simulink model "MRAC_Lab2_Normalizado"  (R2020a)
settings: Solver=VariableStepAuto  StartTime=0.0  StopTime=200  RelTol=1e-3
model workspace (MAT data in the model file):
  gamma = Simulink.Parameter
  gamma.Value = 2
  gamma.DataType = 'auto'
  gamma.Dimensions = [1 1]
  gamma2 = Simulink.Parameter
  gamma2.Value = 0.0005
  gamma2.DataType = 'auto'
  gamma2.Dimensions = [1 1]
undefined symbols (not defined in the file): den, num
settings Model: Creator=Lenovo  LastModifiedBy=Lenovo

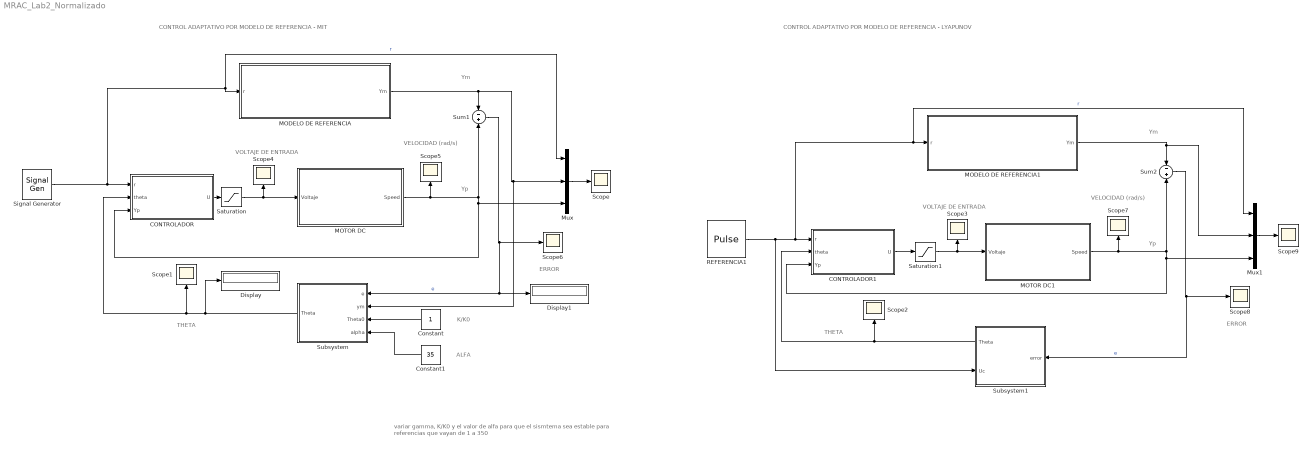
== system MRAC_Lab2_Normalizado ==
  note: variar gamma, K/K0 y el valor de alfa para que el sismtema sea
      | estable para referencias que vayan de 1 a 350
  note: ALFA
  note: K/K0
  note: THETA
  note: VELOCIDAD (rad/s)
  note: Ym
  note: Yp
  note: VOLTAJE DE ENTRADA
  note: ERROR
  note: CONTROL ADAPTATIVO POR MODELO DE REFERENCIA - MIT
  note: THETA
  note: ERROR
  note: Ym
  note: Yp
  note: VELOCIDAD (rad/s)
  note: VOLTAJE DE ENTRADA
  note: CONTROL ADAPTATIVO POR MODELO DE REFERENCIA - LYAPUNOV
  CONTROLADOR : Subsystem
  CONTROLADOR1 : Subsystem
  Constant : Constant
  Constant1 : Constant  Value=35
  Display : Display
  Display1 : Display
  MODELO DE REFERENCIA : Subsystem
  MODELO DE REFERENCIA1 : Subsystem
  MOTOR DC : Subsystem
  MOTOR DC1 : Subsystem
  Mux : Mux  Inputs=3
  Mux1 : Mux  Inputs=3
  REFERENCIA1 : DiscretePulseGenerator  PulseType=Time based  Amplitude=100  Period=20  PulseWidth=50
  Saturation : Saturate  UpperLimit=9  LowerLimit=-9
  Saturation1 : Saturate  UpperLimit=18  LowerLimit=0
  Scope{,1..9} (10 alike) : Scope
  Signal Generator : SignalGenerator  WaveForm=square  Amplitude=50  Frequency=1/40
  Subsystem : Subsystem
  Subsystem1 : Subsystem
      settings: PortSchema="{\"entries\":[{\"content\":{\"sides\":[{\"content\":{\"connectorIds\":[\"In1\"]},\"type\":\"ConnectorPlacement.EquallySpacedRectSide\",\"uuid\":\"f4eaeb92-0652-4579-b232-1e80a6b1a6f8\"},{\"content\":{\"connectorIds\":[\"Out1\",\"In2\"],\"side\":\"RIGHT\"},\"type\":\"ConnectorPlacement.EquallySpacedRectSide\",\"uuid\":\"560fd036-08cc-4dd0-b8b1-11ed0b1d96a0\"},{\"content\":{\"connectorIds\":[],\"side\":\"TOP\"},\"type\":\"ConnectorPlacement.EquallySpacedRectSide\",\"uuid\":\"cc615b19-c919-421a-ac38-f3609e4d576b\"}]},\"type\":\"ConnectorPlacement.EquallySpacedConnector\",\"uuid\":\"33a90cb3-3880-43e0-9034-86a65faaa9ff\"}],\"packageUris\":[\"http://schema.mathworks.com/mf0/Connector/19700101\"],\"version\":\"1.0\"}"
  Sum1 : Sum  Inputs=-|+
  Sum2 : Sum  Inputs=-|+
  wires:
  MODELO DE REFERENCIA/1(Ym) -> Sum1/1, Subsystem/2(ym), Mux/2
  Sum1/1 -> Subsystem/1(e), Display1/1, Scope6/1  "e"
  Mux/1 -> Scope/1
  Subsystem/1(Theta) -> Display/1, Scope1/1, CONTROLADOR/2(theta)
  Signal Generator/1 -> Mux/1, MODELO DE REFERENCIA/1(r), CONTROLADOR/1(r)  "r"
  MOTOR DC/1(Speed) -> Mux/3, CONTROLADOR/3(Yp), Sum1/2, Scope5/1
  Constant/1 -> Subsystem/3(Theta0)
  Constant1/1 -> Subsystem/4(alpha)
  CONTROLADOR/1(U) -> Saturation/1
  Saturation/1 -> MOTOR DC/1(Voltaje), Scope4/1
  Subsystem1/1(Theta) -> CONTROLADOR1/2(theta), Scope2/1
  MOTOR DC1/1(Speed) -> CONTROLADOR1/3(Yp), Mux1/3, Sum2/2, Scope7/1
  CONTROLADOR1/1(U) -> Saturation1/1
  REFERENCIA1/1 -> Subsystem1/2(Uc), CONTROLADOR1/1(r), Mux1/1, MODELO DE REFERENCIA1/1(r)  "r"
  MODELO DE REFERENCIA1/1(Ym) -> Sum2/1, Mux1/2
  Saturation1/1 -> Scope3/1, MOTOR DC1/1(Voltaje)
  Sum2/1 -> Subsystem1/1(error), Scope8/1  "e"
  Mux1/1 -> Scope9/1

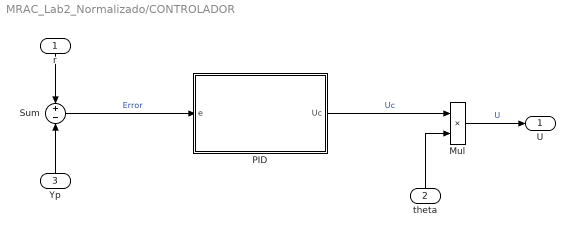
== system MRAC_Lab2_Normalizado/CONTROLADOR ==
  r : Inport
  theta : Inport  Port=2
  Yp : Inport  Port=3
  Mul : Product
  PID : Subsystem
  Sum : Sum  Inputs=+|-
  U : Outport  VectorParamsAs1DForOutWhenUnconnected=off
  wires:
  theta/1 -> Mul/2
  r/1 -> Sum/1
  Yp/1 -> Sum/2
  PID/1(Uc) -> Mul/1  "Uc"
  Sum/1 -> PID/1(e)  "Error"
  Mul/1 -> U/1  "U"

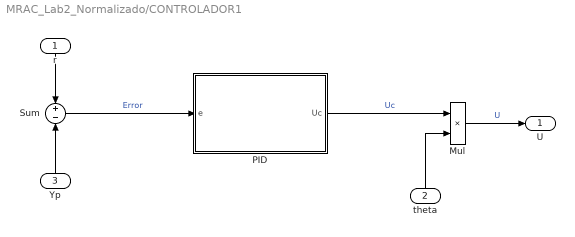
== system MRAC_Lab2_Normalizado/CONTROLADOR1 ==
  r : Inport
  theta : Inport  Port=2
  Yp : Inport  Port=3
  Mul : Product
  PID : Subsystem
  Sum : Sum  Inputs=+|-
  U : Outport  VectorParamsAs1DForOutWhenUnconnected=off
  wires:
  theta/1 -> Mul/2
  r/1 -> Sum/1
  Yp/1 -> Sum/2
  PID/1(Uc) -> Mul/1  "Uc"
  Sum/1 -> PID/1(e)  "Error"
  Mul/1 -> U/1  "U"

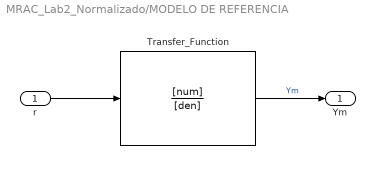
== system MRAC_Lab2_Normalizado/MODELO DE REFERENCIA ==
  r : Inport
  Transfer_Function : TransferFcn  Numerator=[num]  Denominator=[den]
  Ym : Outport  VectorParamsAs1DForOutWhenUnconnected=off
  wires:
  Transfer_Function/1 -> Ym/1  "Ym"
  r/1 -> Transfer_Function/1

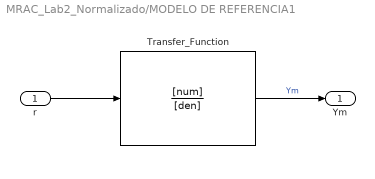
== system MRAC_Lab2_Normalizado/MODELO DE REFERENCIA1 ==
  r : Inport
  Transfer_Function : TransferFcn  Numerator=[num]  Denominator=[den]
  Ym : Outport  VectorParamsAs1DForOutWhenUnconnected=off
  wires:
  Transfer_Function/1 -> Ym/1  "Ym"
  r/1 -> Transfer_Function/1

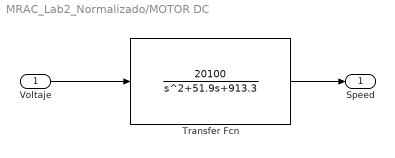
== system MRAC_Lab2_Normalizado/MOTOR DC ==
  Voltaje : Inport
  Transfer Fcn : TransferFcn  Numerator=[20100]  Denominator="[1   51.9  913.3]"
  Speed : Outport
  wires:
  Transfer Fcn/1 -> Speed/1
  Voltaje/1 -> Transfer Fcn/1

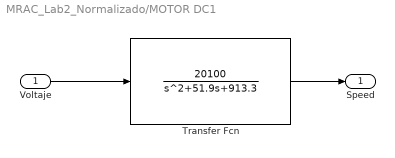
== system MRAC_Lab2_Normalizado/MOTOR DC1 ==
  Voltaje : Inport
  Transfer Fcn : TransferFcn  Numerator=[20100]  Denominator="[1   51.9  913.3]"
  Speed : Outport
  wires:
  Transfer Fcn/1 -> Speed/1
  Voltaje/1 -> Transfer Fcn/1

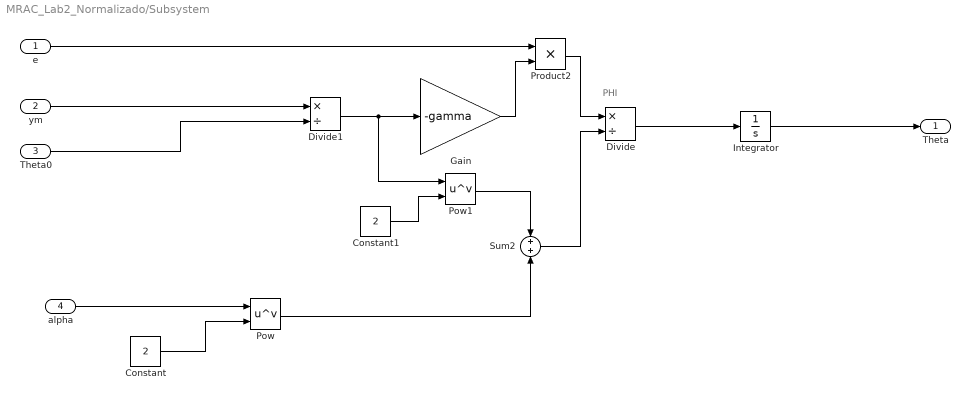
== system MRAC_Lab2_Normalizado/Subsystem ==
  note: PHI
  e : Inport
  ym : Inport  Port=2
  Theta0 : Inport  Port=3
  alpha : Inport  Port=4
  Constant : Constant  Value=2
  Constant1 : Constant  Value=2
  Divide : Product  Inputs=*/  RndMeth=Zero  SaturateOnIntegerOverflow=on
  Divide1 : Product  Inputs=*/  RndMeth=Zero  SaturateOnIntegerOverflow=on
  Gain : Gain  Gain=-gamma
  Integrator : Integrator
  Pow : Math  Operator=pow  SignedPower=on  RndMeth=Zero  SaturateOnIntegerOverflow=on
  Pow1 : Math  Operator=pow  SignedPower=on  RndMeth=Zero  SaturateOnIntegerOverflow=on
  Product2 : Product
  Sum2 : Sum
  Theta : Outport
  wires:
  Divide1/1 -> Pow1/1, Gain/1
  Sum2/1 -> Divide/2
  Pow1/1 -> Sum2/1
  Divide/1 -> Integrator/1
  Integrator/1 -> Theta/1
  Gain/1 -> Product2/2
  Product2/1 -> Divide/1
  e/1 -> Product2/1
  alpha/1 -> Pow/1
  Pow/1 -> Sum2/2
  Constant/1 -> Pow/2
  Constant1/1 -> Pow1/2
  ym/1 -> Divide1/1
  Theta0/1 -> Divide1/2

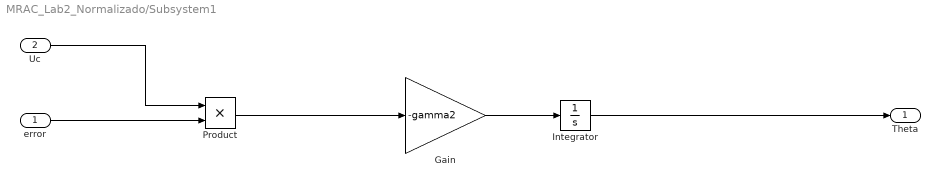
== system MRAC_Lab2_Normalizado/Subsystem1 ==
  error : Inport
  Uc : Inport  Port=2
  Gain : Gain  Gain=-gamma2
  Integrator : Integrator
  Product : Product
  Theta : Outport
  wires:
  Uc/1 -> Product/1
  error/1 -> Product/2
  Product/1 -> Gain/1
  Gain/1 -> Integrator/1
  Integrator/1 -> Theta/1

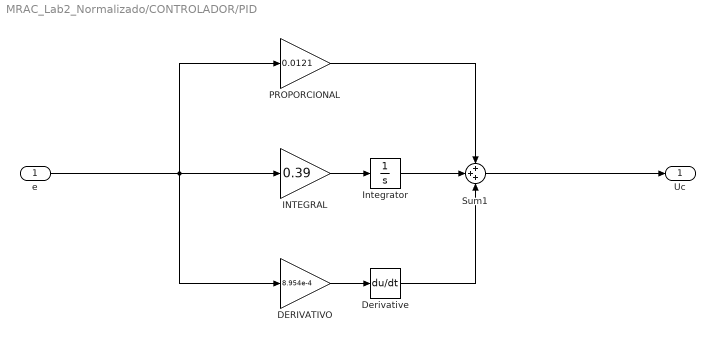
== system MRAC_Lab2_Normalizado/CONTROLADOR/PID ==
  e : Inport
  DERIVATIVO : Gain  Gain=8.954e-4
  Derivative : Derivative
  INTEGRAL : Gain  Gain=0.39
  Integrator : Integrator
  PROPORCIONAL : Gain  Gain=0.0121
  Sum1 : Sum  Inputs=+++
  Uc : Outport
  wires:
  Sum1/1 -> Uc/1
  INTEGRAL/1 -> Integrator/1
  Integrator/1 -> Sum1/2
  e/1 -> DERIVATIVO/1, INTEGRAL/1, PROPORCIONAL/1
  DERIVATIVO/1 -> Derivative/1
  PROPORCIONAL/1 -> Sum1/1
  Derivative/1 -> Sum1/3

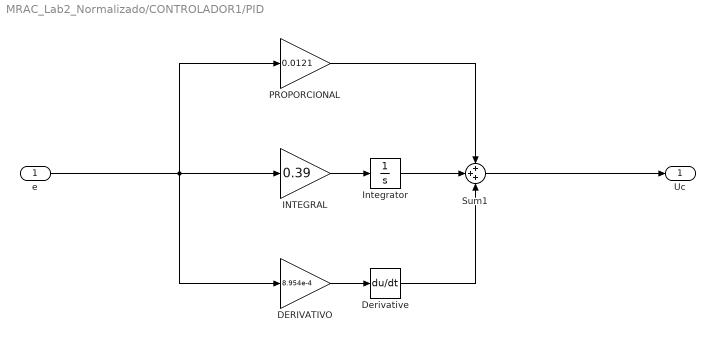
== system MRAC_Lab2_Normalizado/CONTROLADOR1/PID ==
  e : Inport
  DERIVATIVO : Gain  Gain=8.954e-4
  Derivative : Derivative
  INTEGRAL : Gain  Gain=0.39
  Integrator : Integrator
  PROPORCIONAL : Gain  Gain=0.0121
  Sum1 : Sum  Inputs=+++
  Uc : Outport
  wires:
  Sum1/1 -> Uc/1
  INTEGRAL/1 -> Integrator/1
  Integrator/1 -> Sum1/2
  e/1 -> DERIVATIVO/1, INTEGRAL/1, PROPORCIONAL/1
  DERIVATIVO/1 -> Derivative/1
  PROPORCIONAL/1 -> Sum1/1
  Derivative/1 -> Sum1/3
